simulink model "part1_8"  (R2022b)
settings: Solver=VariableStepAuto  StartTime=0.0  StopTime=2  RelTol=1e-3
undefined symbols (not defined in the file or in its folder): den, G, Gc, Gd_matched_T1, Gd_matched_T2, Gd_matched_T3, Gd_tustin_T1, Gd_tustin_T2, Gd_tustin_T3, Gdb, Gdiscrete, gp, Kdd, Kid, Kpd, N1, num, Ts
libraries: simulink x3, slpidlib x2
settings Model: Creator=nimaz  LastModifiedBy=nimaz
settings SolverCC: AlgebraicLoopSolver=TrustRegion
settings DebuggingCC: ArithmeticOperatorsInVariantConditions=warning
settings SFSimCC: CustomCodeUndefinedFunction=UseInterfaceOnly
settings CodeAppCC: StateflowObjectComments=on

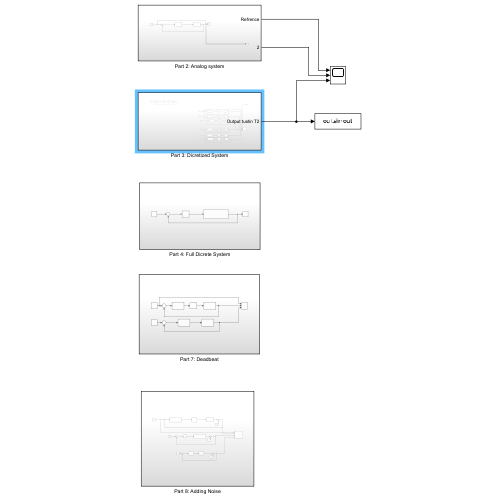
[thumbnail: Simulink's stored preview of the top-level diagram]
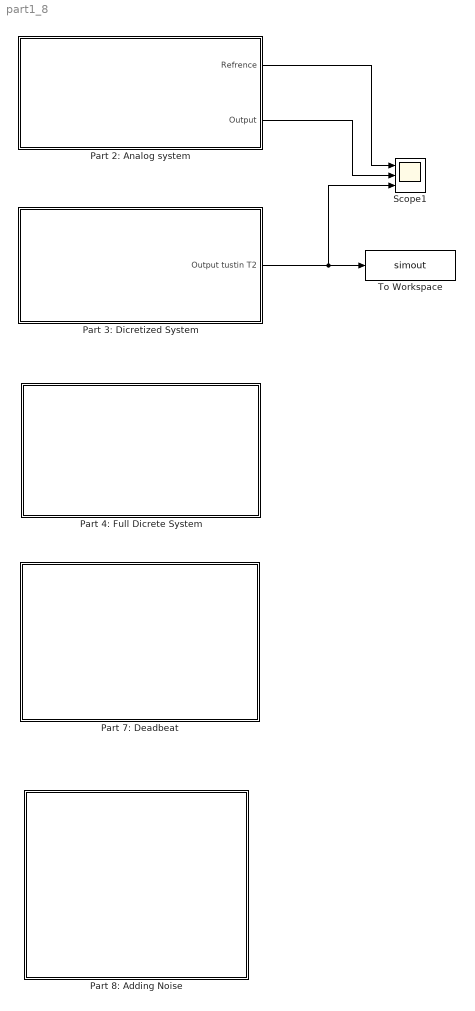
== system part1_8 ==
  Part 2: Analog system : Subsystem
  Part 3: Dicretized System : Subsystem
  Part 4: Full Dicrete System : Subsystem
  Part 7: Deadbeat : Subsystem
  Part 8: Adding Noise : Subsystem
  Scope1 : Scope  NumInputPorts=3
  To Workspace : ToWorkspace  VariableName=simout  SaveFormat=Timeseries  SampleTime=-1
  wires:
  Part 2: Analog system/1(Refrence) -> Scope1/1
  Part 2: Analog system/2(Output) -> Scope1/2
  Part 3: Dicretized System/1(Output tustin T2) -> To Workspace/1, Scope1/3

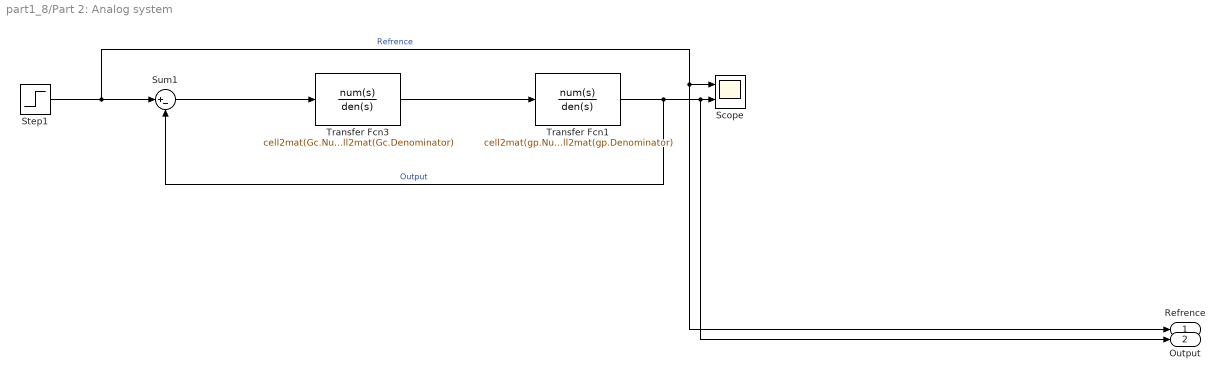
== system part1_8/Part 2: Analog system ==
  Scope : Scope  NumInputPorts=2
  Step1 : Step  Time=0  SampleTime=0
  Sum1 : Sum  Inputs=|+-
  Transfer Fcn1 : TransferFcn  Numerator=cell2mat(gp.Numerator)  Denominator=cell2mat(gp.Denominator)
  Transfer Fcn3 : TransferFcn  Numerator=cell2mat(Gc.Numerator)  Denominator=cell2mat(Gc.Denominator)
  Refrence : Outport
  Output : Outport  Port=2
  wires:
  Transfer Fcn3/1 -> Transfer Fcn1/1
  Sum1/1 -> Transfer Fcn3/1
  Step1/1 -> Refrence/1, Scope/1, Sum1/1  "Refrence"
  Transfer Fcn1/1 -> Sum1/2, Output/1, Scope/2  "Output"

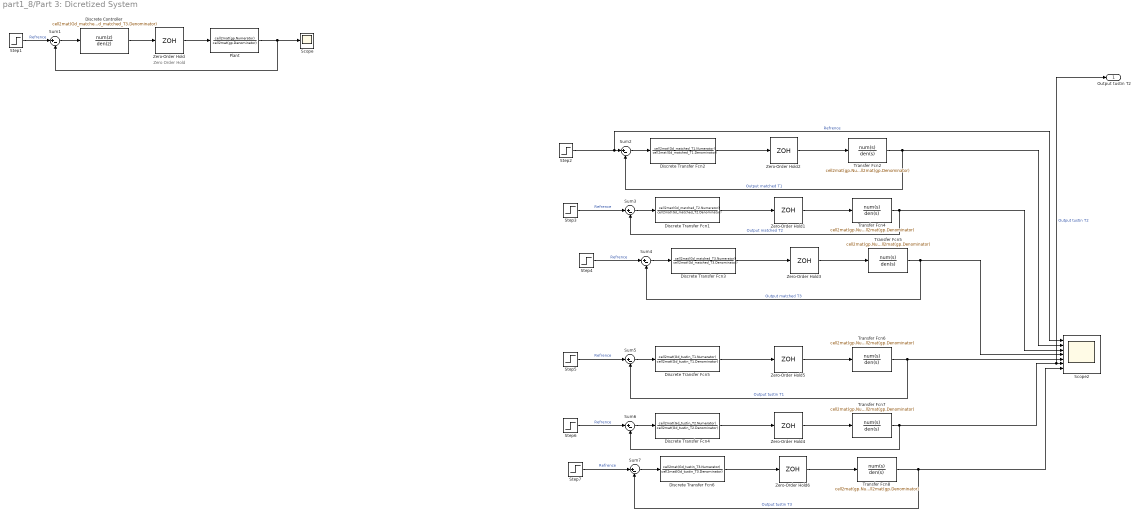
== system part1_8/Part 3: Dicretized System ==
  note: Zero Order Hold
  Discrete Transfer Fcn1 : DiscreteTransferFcn  Numerator=cell2mat(Gd_matched_T2.Numerator)  Denominator=cell2mat(Gd_matched_T2.Denominator)  SampleTime=Ts(2)
  Discrete Transfer Fcn2 : DiscreteTransferFcn  Numerator=cell2mat(Gd_matched_T1.Numerator)  Denominator=cell2mat(Gd_matched_T1.Denominator)  SampleTime=Ts(1)
  Discrete Transfer Fcn3 : DiscreteTransferFcn  Numerator=cell2mat(Gd_matched_T3.Numerator)  Denominator=cell2mat(Gd_matched_T3.Denominator)  SampleTime=Ts(3)
  Discrete Transfer Fcn4 : DiscreteTransferFcn  Numerator=cell2mat(Gd_tustin_T2.Numerator)  Denominator=cell2mat(Gd_tustin_T2.Denominator)  SampleTime=Ts(2)
  Discrete Transfer Fcn5 : DiscreteTransferFcn  Numerator=cell2mat(Gd_tustin_T1.Numerator)  Denominator=cell2mat(Gd_tustin_T1.Denominator)  SampleTime=Ts(1)
  Discrete Transfer Fcn6 : DiscreteTransferFcn  Numerator=cell2mat(Gd_tustin_T3.Numerator)  Denominator=cell2mat(Gd_tustin_T3.Denominator)  SampleTime=Ts(3)
  Discrete Controller : DiscreteTransferFcn  Numerator=cell2mat(Gd_matched_T3.Numerator)  Denominator=cell2mat(Gd_matched_T3.Denominator)  SampleTime=Ts(3)
  Plant : TransferFcn  Numerator=cell2mat(gp.Numerator)  Denominator=cell2mat(gp.Denominator)
  Scope : Scope
  Scope2 : Scope  NumInputPorts=7
  Step{1..7} (7 alike) : Step  Time=0  SampleTime=0
  Sum{1..7} (7 alike) : Sum  Inputs=|+-
  Transfer Fcn{2,4..8} (6 alike) : TransferFcn  Numerator=cell2mat(gp.Numerator)  Denominator=cell2mat(gp.Denominator)
  Zero-Order Hold1 : ZeroOrderHold  SampleTime=Ts(2)
  Zero-Order Hold2 : ZeroOrderHold  SampleTime=Ts(1)
  Zero-Order Hold3 : ZeroOrderHold  SampleTime=Ts(3)
  Zero-Order Hold4 : ZeroOrderHold  SampleTime=Ts(2)
  Zero-Order Hold5 : ZeroOrderHold  SampleTime=Ts(1)
  Zero-Order Hold6 : ZeroOrderHold  SampleTime=Ts(3)
  Zero-Order Hold : ZeroOrderHold  SampleTime=Ts(3)
  Output tustin T2 : Outport
  wires:
  Transfer Fcn7/1 -> Output tustin T2/1, Scope2/6, Sum6/2  "Output tustin T2"
  Discrete Transfer Fcn4/1 -> Zero-Order Hold4/1
  Transfer Fcn8/1 -> Scope2/7, Sum7/2  "Output tustin T3"
  Transfer Fcn6/1 -> Sum5/2, Scope2/5  "Output tustin T1"
  Sum2/1 -> Discrete Transfer Fcn2/1
  Sum6/1 -> Discrete Transfer Fcn4/1
  Transfer Fcn5/1 -> Sum4/2, Scope2/4  "Output matched T3"
  Step6/1 -> Sum6/1  "Refrence"
  Discrete Transfer Fcn6/1 -> Zero-Order Hold6/1
  Zero-Order Hold4/1 -> Transfer Fcn7/1
  Discrete Transfer Fcn2/1 -> Zero-Order Hold2/1
  Zero-Order Hold5/1 -> Transfer Fcn6/1
  Transfer Fcn4/1 -> Sum3/2, Scope2/3  "Output matched T2"
  Discrete Transfer Fcn5/1 -> Zero-Order Hold5/1
  Discrete Transfer Fcn3/1 -> Zero-Order Hold3/1
  Step2/1 -> Scope2/1, Sum2/1  "Refrence"
  Sum7/1 -> Discrete Transfer Fcn6/1
  Zero-Order Hold6/1 -> Transfer Fcn8/1
  Transfer Fcn2/1 -> Sum2/2, Scope2/2  "Output matched T1"
  Sum3/1 -> Discrete Transfer Fcn1/1
  Step7/1 -> Sum7/1  "Refrence"
  Step5/1 -> Sum5/1  "Refrence"
  Sum5/1 -> Discrete Transfer Fcn5/1
  Zero-Order Hold2/1 -> Transfer Fcn2/1
  Sum4/1 -> Discrete Transfer Fcn3/1
  Step4/1 -> Sum4/1  "Refrence"
  Zero-Order Hold3/1 -> Transfer Fcn5/1
  Discrete Transfer Fcn1/1 -> Zero-Order Hold1/1
  Step3/1 -> Sum3/1  "Refrence"
  Zero-Order Hold1/1 -> Transfer Fcn4/1
  Discrete Controller/1 -> Zero-Order Hold/1
  Zero-Order Hold/1 -> Plant/1
  Sum1/1 -> Discrete Controller/1
  Step1/1 -> Sum1/1  "Refrence"
  Plant/1 -> Sum1/2, Scope/1

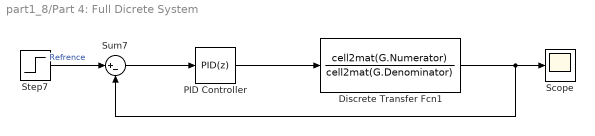
== system part1_8/Part 4: Full Dicrete System ==
  Discrete Transfer Fcn1 : DiscreteTransferFcn  Numerator=cell2mat(G.Numerator)  Denominator=cell2mat(G.Denominator)  SampleTime=Ts(2)
  PID Controller : slpidlib/PID Controller  Controller=PID  Form=Parallel  TimeDomain=Discrete-time  UseExternalTs=off  SampleTime=Ts(2)  IntegratorMethod=Forward Euler  FilterMethod=Forward Euler  ControllerParametersSource=internal  P=Kpd  I=Kid  UseKiTs=off  D=Kdd  N=N1  UseFilter=on  TunerSelectOption=Transfer Function Based (PID Tuner App)  InitialConditionSource=internal  InitialConditionForIntegrator=0  InitialConditionForFilter=0  DifferentiatorICPrevScaledInput=0  ExternalReset=none  TrackingMode=off  Kt=1  LimitOutput=off  SatLimitsSource=internal  UpperSaturationLimit=inf  LowerSaturationLimit=-inf  LinearizeAsGain=on  AntiWindupMode=none  Kb=1  LimitIntegrator=off  UpperIntegratorSaturationLimit=inf  LowerIntegratorSaturationLimit=-inf  POutMin=[]  POutMax=[]  IOutMin=[]  IOutMax=[]  DOutMin=[]  DOutMax=[]  NOutMin=[]  NOutMax=[]  SumOutMin=[]  SumOutMax=[]  SaturationOutMin=[]  SaturationOutMax=[]  PParamMin=[]  PParamMax=[]  IParamMin=[]  IParamMax=[]  DParamMin=[]  DParamMax=[]  NParamMin=[]  NParamMax=[]  KbParamMin=[]  KbParamMax=[]  KtParamMin=[]  KtParamMax=[]  KbOutMin=[]  KbOutMax=[]  KtOutMin=[]  KtOutMax=[]  IntegratorOutMin=[]  IntegratorOutMax=[]  FilterOutMin=[]  FilterOutMax=[]  SumI1OutMin=[]  SumI1OutMax=[]  SumI2OutMin=[]  SumI2OutMax=[]  SumI3OutMin=[]  SumI3OutMax=[]  SumI4OutMin=[]  SumI4OutMax=[]  SumDOutMin=[]  SumDOutMax=[]  DifferentiatorOutMin=[]  DifferentiatorOutMax=[]  FilterDiffOutCoefMin=[]  FilterDiffOutCoefMax=[]  ReciprocalOutMin=[]  ReciprocalOutMax=[]  SumDenOutMin=[]  SumDenOutMax=[]  SumNumOutMin=[]  SumNumOutMax=[]  DivideOutMin=[]  DivideOutMax=[]  UdiffTsProdOutMin=[]  UdiffTsProdOutMax=[]  NTsProdOutMin=[]  NTsProdOutMax=[]  UintegralTsProdOutMin=[]  UintegralTsProdOutMax=[]  UngainTsProdOutMin=[]  UngainTsProdOutMax=[]  ClampingZeroOutDataTypeStr=Inherit: Inherit via back propagation  ClampingZeroOutMin=[]  ClampingZeroOutMax=[]  FilterDenConstantOutDataTypeStr=Inherit: Inherit via back propagation  FilterDenConstantOutMin=[]  FilterDenConstantOutMax=[]  PCopyOutDataTypeStr=Inherit: Inherit via back propagation  PCopyOutMin=[]  PCopyOutMax=[]  NCopyOutDataTypeStr=Inherit: Inherit via back propagation  NCopyOutMin=[]  NCopyOutMax=[]  IntegratorContinuousStateAttributes=''  IntegratorStateMustResolveToSignalObject=off  IntegratorRTWStateStorageClass=Auto  FilterContinuousStateAttributes=''  FilterStateMustResolveToSignalObject=off  FilterRTWStateStorageClass=Auto  ParallelPVariant=InternalParameters  IdealPVariant=Disabled  IVariant=InternalParameters  DVariant=InternalParameters  IntegratorVariant=Discrete  SatVariant=Disabled  AWVariant=Passthrough  PCopyVariant=Disabled  TRVariant=Disabled  FdbkBlocksVariant=Forward  IdealPFdbkVariant=Disabled  SatFdbkVariant=Disabled  DerivativeFilterVariant=ForwardEulerFilter  NVariant=InternalParameters  NCopyVariant=Disabled  FilterICVariant=InternalICsFilter  IntegratorICVariant=InternalICs  ExternalResetVariant=Disabled  TRSumVariant=Passthrough  SumFdbkVariant=Disabled  SumVariant=Sum_PID  TsampFilterVariant=InternalTs  TsampNgainVariant=Passthrough  TsampIntegralVariant=Passthrough  ExternalSaturationOutDataTypeStr=Inherit: Same as second input
  Scope : Scope
  Step7 : Step  Time=0  SampleTime=0
  Sum7 : Sum  Inputs=|+-
  wires:
  Discrete Transfer Fcn1/1 -> Scope/1, Sum7/2
  Sum7/1 -> PID Controller/1
  Step7/1 -> Sum7/1  "Refrence"
  PID Controller/1 -> Discrete Transfer Fcn1/1

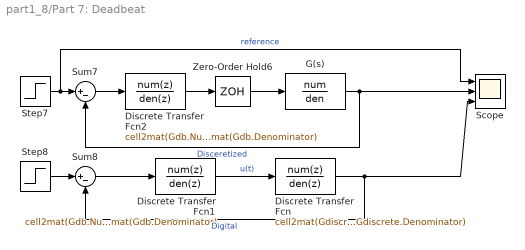
== system part1_8/Part 7: Deadbeat ==
  Discrete Transfer Fcn : DiscreteTransferFcn  Numerator=cell2mat(Gdiscrete.Numerator)  Denominator=cell2mat(Gdiscrete.Denominator)  SampleTime=Ts(2)
  Discrete Transfer Fcn1 : DiscreteTransferFcn  Numerator=cell2mat(Gdb.Numerator)  Denominator=cell2mat(Gdb.Denominator)  SampleTime=Ts(2)
  Discrete Transfer Fcn2 : DiscreteTransferFcn  Numerator=cell2mat(Gdb.Numerator)  Denominator=cell2mat(Gdb.Denominator)  SampleTime=Ts(2)
  G(s) : TransferFcn  Numerator=num  Denominator=den
  Scope : Scope  NumInputPorts=3
  Step7 : Step  Time=0  SampleTime=0
  Step8 : Step  Time=0  SampleTime=0
  Sum7 : Sum  Inputs=|+-
  Sum8 : Sum  Inputs=|+-
  Zero-Order Hold6 : ZeroOrderHold  SampleTime=Ts(2)
  wires:
  G(s)/1 -> Sum7/2, Scope/2  "Disceretized"
  Step7/1 -> Scope/1, Sum7/1  "reference"
  Step8/1 -> Sum8/1
  Discrete Transfer Fcn/1 -> Scope/3, Sum8/2  "Digital"
  Sum7/1 -> Discrete Transfer Fcn2/1
  Zero-Order Hold6/1 -> G(s)/1
  Discrete Transfer Fcn2/1 -> Zero-Order Hold6/1
  Discrete Transfer Fcn1/1 -> Discrete Transfer Fcn/1  "u(t)"
  Sum8/1 -> Discrete Transfer Fcn1/1

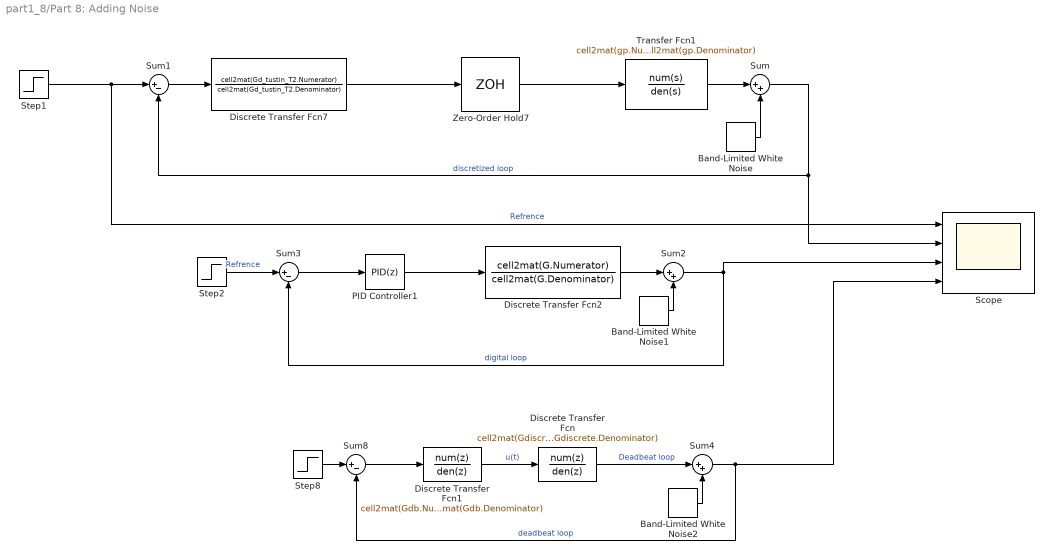
== system part1_8/Part 8: Adding Noise ==
  Band-Limited White Noise : simulink/Sources/Band-Limited White Noise  Cov=1e-5  Ts=Ts(2)  seed=[23341]
  Band-Limited White Noise1 : simulink/Sources/Band-Limited White Noise  Cov=1e-5  Ts=Ts(2)  seed=[23341]
  Band-Limited White Noise2 : simulink/Sources/Band-Limited White Noise  Cov=1e-5  Ts=Ts(2)  seed=[23341]
  Discrete Transfer Fcn : DiscreteTransferFcn  Numerator=cell2mat(Gdiscrete.Numerator)  Denominator=cell2mat(Gdiscrete.Denominator)  SampleTime=Ts(2)
  Discrete Transfer Fcn1 : DiscreteTransferFcn  Numerator=cell2mat(Gdb.Numerator)  Denominator=cell2mat(Gdb.Denominator)  SampleTime=Ts(2)
  Discrete Transfer Fcn2 : DiscreteTransferFcn  Numerator=cell2mat(G.Numerator)  Denominator=cell2mat(G.Denominator)  SampleTime=Ts(2)
  Discrete Transfer Fcn7 : DiscreteTransferFcn  Numerator=cell2mat(Gd_tustin_T2.Numerator)  Denominator=cell2mat(Gd_tustin_T2.Denominator)  SampleTime=Ts(2)
  PID Controller1 : slpidlib/PID Controller  Controller=PID  Form=Parallel  TimeDomain=Discrete-time  UseExternalTs=off  SampleTime=Ts(2)  IntegratorMethod=Forward Euler  FilterMethod=Forward Euler  ControllerParametersSource=internal  P=Kpd  I=Kid  UseKiTs=off  D=Kdd  N=N1  UseFilter=on  TunerSelectOption=Transfer Function Based (PID Tuner App)  InitialConditionSource=internal  InitialConditionForIntegrator=0  InitialConditionForFilter=0  DifferentiatorICPrevScaledInput=0  ExternalReset=none  TrackingMode=off  Kt=1  LimitOutput=off  SatLimitsSource=internal  UpperSaturationLimit=inf  LowerSaturationLimit=-inf  LinearizeAsGain=on  AntiWindupMode=none  Kb=1  LimitIntegrator=off  UpperIntegratorSaturationLimit=inf  LowerIntegratorSaturationLimit=-inf  POutMin=[]  POutMax=[]  IOutMin=[]  IOutMax=[]  DOutMin=[]  DOutMax=[]  NOutMin=[]  NOutMax=[]  SumOutMin=[]  SumOutMax=[]  SaturationOutMin=[]  SaturationOutMax=[]  PParamMin=[]  PParamMax=[]  IParamMin=[]  IParamMax=[]  DParamMin=[]  DParamMax=[]  NParamMin=[]  NParamMax=[]  KbParamMin=[]  KbParamMax=[]  KtParamMin=[]  KtParamMax=[]  KbOutMin=[]  KbOutMax=[]  KtOutMin=[]  KtOutMax=[]  IntegratorOutMin=[]  IntegratorOutMax=[]  FilterOutMin=[]  FilterOutMax=[]  SumI1OutMin=[]  SumI1OutMax=[]  SumI2OutMin=[]  SumI2OutMax=[]  SumI3OutMin=[]  SumI3OutMax=[]  SumI4OutMin=[]  SumI4OutMax=[]  SumDOutMin=[]  SumDOutMax=[]  DifferentiatorOutMin=[]  DifferentiatorOutMax=[]  FilterDiffOutCoefMin=[]  FilterDiffOutCoefMax=[]  ReciprocalOutMin=[]  ReciprocalOutMax=[]  SumDenOutMin=[]  SumDenOutMax=[]  SumNumOutMin=[]  SumNumOutMax=[]  DivideOutMin=[]  DivideOutMax=[]  UdiffTsProdOutMin=[]  UdiffTsProdOutMax=[]  NTsProdOutMin=[]  NTsProdOutMax=[]  UintegralTsProdOutMin=[]  UintegralTsProdOutMax=[]  UngainTsProdOutMin=[]  UngainTsProdOutMax=[]  ClampingZeroOutDataTypeStr=Inherit: Inherit via back propagation  ClampingZeroOutMin=[]  ClampingZeroOutMax=[]  FilterDenConstantOutDataTypeStr=Inherit: Inherit via back propagation  FilterDenConstantOutMin=[]  FilterDenConstantOutMax=[]  PCopyOutDataTypeStr=Inherit: Inherit via back propagation  PCopyOutMin=[]  PCopyOutMax=[]  NCopyOutDataTypeStr=Inherit: Inherit via back propagation  NCopyOutMin=[]  NCopyOutMax=[]  IntegratorContinuousStateAttributes=''  IntegratorStateMustResolveToSignalObject=off  IntegratorRTWStateStorageClass=Auto  FilterContinuousStateAttributes=''  FilterStateMustResolveToSignalObject=off  FilterRTWStateStorageClass=Auto  ParallelPVariant=InternalParameters  IdealPVariant=Disabled  IVariant=InternalParameters  DVariant=InternalParameters  IntegratorVariant=Discrete  SatVariant=Disabled  AWVariant=Passthrough  PCopyVariant=Disabled  TRVariant=Disabled  FdbkBlocksVariant=Forward  IdealPFdbkVariant=Disabled  SatFdbkVariant=Disabled  DerivativeFilterVariant=ForwardEulerFilter  NVariant=InternalParameters  NCopyVariant=Disabled  FilterICVariant=InternalICsFilter  IntegratorICVariant=InternalICs  ExternalResetVariant=Disabled  TRSumVariant=Passthrough  SumFdbkVariant=Disabled  SumVariant=Sum_PID  TsampFilterVariant=InternalTs  TsampNgainVariant=Passthrough  TsampIntegralVariant=Passthrough  ExternalSaturationOutDataTypeStr=Inherit: Same as second input
  Scope : Scope  NumInputPorts=4
  Step1 : Step  Time=0  SampleTime=0
  Step2 : Step  Time=0  SampleTime=0
  Step8 : Step  Time=0  SampleTime=0
  Sum : Sum  Inputs=|++
  Sum1 : Sum  Inputs=|+-
  Sum2 : Sum  Inputs=|++
  Sum3 : Sum  Inputs=|+-
  Sum4 : Sum  Inputs=|++
  Sum8 : Sum  Inputs=|+-
  Transfer Fcn1 : TransferFcn  Numerator=cell2mat(gp.Numerator)  Denominator=cell2mat(gp.Denominator)
  Zero-Order Hold7 : ZeroOrderHold  SampleTime=Ts(2)
  wires:
  Step2/1 -> Sum3/1  "Refrence"
  Step1/1 -> Scope/1, Sum1/1  "Refrence"
  Sum2/1 -> Sum3/2, Scope/3  "digital loop"
  PID Controller1/1 -> Discrete Transfer Fcn2/1
  Band-Limited White Noise1/1 -> Sum2/2
  Sum3/1 -> PID Controller1/1
  Sum/1 -> Scope/2, Sum1/2  "discretized loop"
  Discrete Transfer Fcn2/1 -> Sum2/1
  Sum1/1 -> Discrete Transfer Fcn7/1
  Transfer Fcn1/1 -> Sum/1
  Band-Limited White Noise/1 -> Sum/2
  Zero-Order Hold7/1 -> Transfer Fcn1/1
  Discrete Transfer Fcn7/1 -> Zero-Order Hold7/1
  Discrete Transfer Fcn1/1 -> Discrete Transfer Fcn/1  "u(t)"
  Discrete Transfer Fcn/1 -> Sum4/1  "Deadbeat loop"
  Step8/1 -> Sum8/1
  Sum8/1 -> Discrete Transfer Fcn1/1
  Band-Limited White Noise2/1 -> Sum4/2
  Sum4/1 -> Scope/4, Sum8/2  "deadbeat loop"
